simulink model "neckVel"  (Simulink 8.0)
settings: Solver=FixedStepDiscrete  StartTime=0.0  StopTime=inf  FixedStep=Ts  RelTol=1e-3
InitFcn:
  | initBalancingController;
values from neighbouring files (symbols this model uses):
  Gains = [  70    0   0  4]    [initNeckVel.m]
  Impedances = [kImpTorso,kImpArms,kImpArms,kImpLegs,kImpLegs]    [initNeckVel.m]
  Rf = [R, zeros(3,3); zeros(3,3), R]    [initNeckVel.m]
  Ts = 0.01    [initBalancingOptTauQpExtWrenches.m]    (also in initNeckVel.m)
undefined symbols (not defined in the file or in its folder): DiscIntNeverNeededParam
libraries: WBCLibrary x35, simulink x2, dspsigops x2
settings Model: Creator=daniele  LastModifiedBy=daniele
settings DebuggingCC: FcnCallInpInsideContextMsg=EnableAllAsWarning
settings CodeAppCC: CustomSymbolStrType=$N$R$M_T
settings GRTTargetCC: CodeReplacementLibrary=C89/C90 (ANSI)  CombineOutputUpdateFcns=off  GRTInterface=on

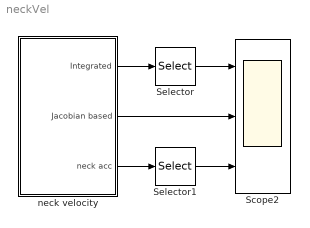
== system neckVel ==
  Scope2 : Scope  NumInputPorts=3
      settings: ShowLegends=on  YMin=-10~-0.035~-0.07  YMax=80~0.04~0.045  SaveName=ScopeData2
  Selector : Selector  InputPortWidth=6  IndexOptions=Index vector (dialog)  Indices=[1:3]  OutputSizes=1
  Selector1 : Selector  InputPortWidth=6  IndexOptions=Index vector (dialog)  Indices=[1:3]  OutputSizes=1
  neck velocity : Subsystem  mask{robotName='iCubGenova01', localName='simulink', Ts=Ts}
      mask prompts: robotName "Robot name"; localName "Local name"
  wires:
  neck velocity/1(Integrated) -> Selector/1
  neck velocity/2(Jacobian based) -> Scope2/2
  Selector/1 -> Scope2/1
  neck velocity/3(neck acc) -> Selector1/1
  Selector1/1 -> Scope2/3

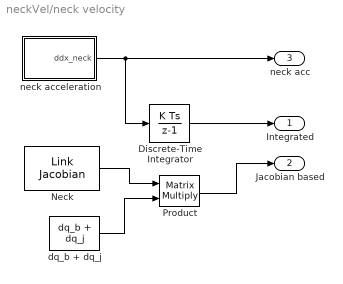
== system neckVel/neck velocity ==
  Discrete-Time Integrator : DiscreteIntegrator  InitialCondition=[0 0 0 0 0 0]  SampleTime=Ts  ICPrevOutput=DiscIntNeverNeededParam  ICPrevScaledInput=DiscIntNeverNeededParam
  Neck : WBCLibrary/wholeBodyModel/Jacobians/Link Jacobian  robotname=robotName  localname=localName  link=chest
  Product : Product  Multiplication=Matrix(*)  SampleTime=Ts  RndMeth=Zero
  dq_b + dq_j : WBCLibrary/wholeBodyStates/dq_b + dq_j  robotName=robotName  localName=localName  Ts=Ts
  neck acceleration : Subsystem  mask{robotName=robotName, localName=localName, Ts=0.010}
      mask prompts: robotName "Robot name"; localName "Local name"
  Integrated : Outport
  Jacobian based : Outport  Port=2
  neck acc : Outport  Port=3
  wires:
  dq_b + dq_j/1 -> Product/2
  Neck/1 -> Product/1
  Product/1 -> Jacobian based/1
  neck acceleration/1(ddx_neck) -> neck acc/1, Discrete-Time Integrator/1
  Discrete-Time Integrator/1 -> Integrated/1

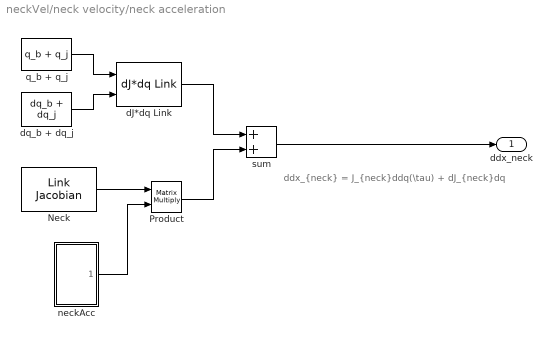
== system neckVel/neck velocity/neck acceleration ==
  note: ddx_{neck} = J_{neck}ddq(\tau) + dJ_{neck}dq
  Neck : WBCLibrary/wholeBodyModel/Jacobians/Link Jacobian  robotname=robotName  localname=localName  link=l_sole
  Product : Product  Multiplication=Matrix(*)  RndMeth=Zero
  dJ*dq Link : WBCLibrary/wholeBodyModel/Dynamics/dJ*dq Link  val=19  robotName=robotName  localName=localName  link=l_sole
  dq_b + dq_j : WBCLibrary/wholeBodyStates/dq_b + dq_j  robotName=robotName  localName=localName  Ts=Ts
  neckAcc : Subsystem  mask{robotName=robotName, Ts=Ts, localName=localName}
      mask prompts: robotName "robot name"; localName "module name"
  q_b + q_j : WBCLibrary/wholeBodyStates/q_b + q_j  robotName=robotName  localName=localName  Ts=Ts
  sum : Sum  SampleTime=Ts
  ddx_neck : Outport
  wires:
  dJ*dq Link/1 -> sum/1
  sum/1 -> ddx_neck/1
  q_b + q_j/1 -> dJ*dq Link/1
  neckAcc/1(ddq(tau)) -> Product/2
  Product/1 -> sum/2
  Neck/1 -> Product/1
  dq_b + dq_j/1 -> dJ*dq Link/2

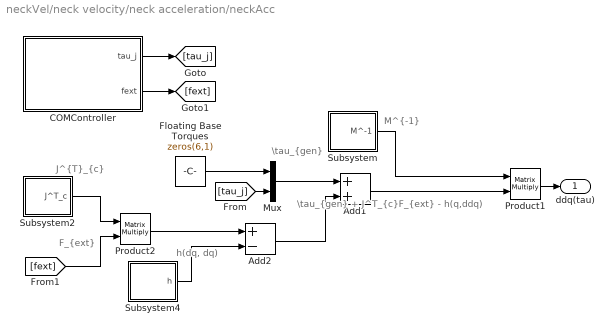
== system neckVel/neck velocity/neck acceleration/neckAcc ==
  note: \tau_{gen} + J^T_{c}F_{ext} - h(q,ddq)
  note: h(dq, dq)
  note: J^{T}_{c}
  note: M^{-1}
  note: F_{ext}
  note: \tau_{gen}
  Add1 : Sum  SampleTime=Ts
  Add2 : Sum  Inputs=+-  SampleTime=Ts
  COMController : Subsystem
  Floating Base Torques : Constant  Value=zeros(6,1)  SampleTime=Ts
  Mux : Mux  Inputs=2
  Product1 : Product  Multiplication=Matrix(*)  SampleTime=Ts
  Product2 : Product  Multiplication=Matrix(*)  SampleTime=Ts
  Subsystem : Subsystem
  Subsystem2 : Subsystem
  Subsystem4 : Subsystem
  ddq(tau) : Outport
  wires:
  Subsystem2/1(J^T_c) -> Product2/1
  [fext] -> Product2/2
  Product2/1 -> Add2/1
  Product1/1 -> ddq(tau)/1
  Add2/1 -> Add1/2
  Subsystem/1(M^-1) -> Product1/1
  Subsystem4/1(h) -> Add2/2
  Add1/1 -> Product1/2
  COMController/1(tau_j) -> [tau_j]
  COMController/2(fext) -> [fext]
  Floating Base Torques/1 -> Mux/1
  [tau_j] -> Mux/2
  Mux/1 -> Add1/1

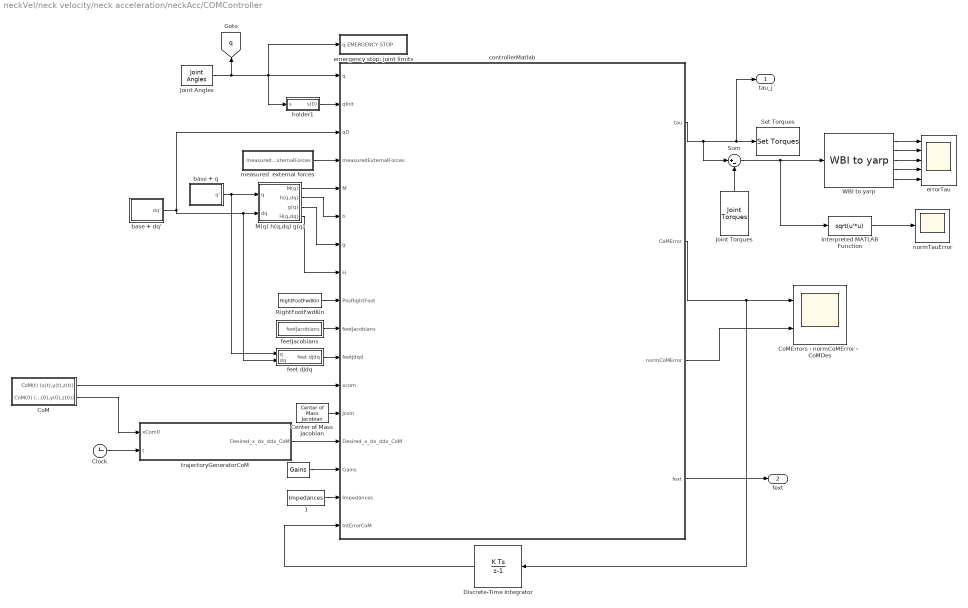
== system neckVel/neck velocity/neck acceleration/neckAcc/COMController ==
  "    " : Constant  Value=Gains
  "    1" : Constant  Value=Impedances
  Center of Mass Jacobian : WBCLibrary/wholeBodyModel/Jacobians/Center of Mass Jacobian  robotName=robotName  localName=localName
  Clock : Clock
  "CoM " : Subsystem
  "CoMErrors - normCoMError -   CoMDes " : Scope  NumInputPorts=2
      settings: ShowLegends=on  TimeRange=35  YMin=-0.1~0  YMax=0.04000000000000001~0.007  SaveName=CoMErrors
  Discrete-Time Integrator : DiscreteIntegrator  InitialCondition=[0 0 0]  SampleTime=Ts  ICPrevOutput=DiscIntNeverNeededParam  ICPrevScaledInput=DiscIntNeverNeededParam
  Interpreted MATLAB Function : MATLABFcn  MATLABFcn=sqrt(u'*u)
  Joint Angles : WBCLibrary/wholeBodyStates/Joint Angles  robotName=robotName  localName=localName
  Joint Torques : WBCLibrary/wholeBodyStates/Joint Torques  robotName=robotName  localName=localName
  M(q) h(q,dq) g(q) : Subsystem
  RightFootFwdKin : WBCLibrary/wholeBodyModel/Forward Kinematics/RightFootFwdKin  robotName=robotName  localName=localName
  Set Torques : WBCLibrary/wholeBodyActuators/Set Torques  val=6  robotName=robotName  localName=localName
  Sum : Sum  Inputs=|+-
  WBI to yarp : WBCLibrary/Utilities/WBI to yarp
  base + dq' : Subsystem
  base + q : Subsystem
  controllerMatlab : MATLAB Function  TreatAsAtomicUnit=on
  emergency stop: joint limits : Subsystem
  errorTau : Scope  NumInputPorts=5
      settings: TimeRange=20  YMin=-12~-5~-5~-5~-5  YMax=6~5~5~5~5
  feet dJdq : Subsystem
  feetJacobians : Subsystem
  holder1 : Subsystem
  measured  external forces : Subsystem
  normTauError : Scope
      settings: TimeRange=80  YMin=0  YMax=60  SaveName=normTauError
  trajectoryGeneratorCoM : MATLAB Function  TreatAsAtomicUnit=on
  tau_j : Outport
  fext : Outport  Port=2
  tag scope: q=global
  wires:
  "    "/1 -> controllerMatlab/15(Gains)
  trajectoryGeneratorCoM/1(Desired_x_dx_ddx_CoM) -> controllerMatlab/14(Desired_x_dx_ddx_CoM)
  Clock/1 -> trajectoryGeneratorCoM/2(t)
  "CoM "/2(CoM(0) (x(0),y(0),z(0))) -> trajectoryGeneratorCoM/1(xCom0)
  RightFootFwdKin/1 -> controllerMatlab/9(PosRightFoot)
  Discrete-Time Integrator/1 -> controllerMatlab/17(IntErrorCoM)
  base + q/1(q') -> feet dJdq/1(q), M(q) h(q,dq) g(q)/1(q)
  base + dq'/1(dq') -> feet dJdq/2(dq), M(q) h(q,dq) g(q)/2(dq), controllerMatlab/3(qD)
  Joint Angles/1 -> [q], emergency stop: joint limits/1(q EMERGENCY STOP), holder1/1(s), controllerMatlab/1(q)
  controllerMatlab/2(CoMError) -> Discrete-Time Integrator/1, "CoMErrors - normCoMError -   CoMDes "/1
  controllerMatlab/3(normCoMError) -> "CoMErrors - normCoMError -   CoMDes "/2
  "    1"/1 -> controllerMatlab/16(Impedances)
  measured  external forces/1(measuredExternalForces) -> controllerMatlab/4(measuredExternalForces)
  Joint Torques/1 -> Sum/2
  Interpreted MATLAB Function/1 -> normTauError/1
  Sum/1 -> WBI to yarp/1, Interpreted MATLAB Function/1
  WBI to yarp/1 -> errorTau/1
  WBI to yarp/2 -> errorTau/2
  WBI to yarp/3 -> errorTau/3
  WBI to yarp/4 -> errorTau/4
  WBI to yarp/5 -> errorTau/5
  M(q) h(q,dq) g(q)/1(M(q)) -> controllerMatlab/5(M)
  M(q) h(q,dq) g(q)/2(h(q,dq)) -> controllerMatlab/6(h)
  M(q) h(q,dq) g(q)/3(g(q)) -> controllerMatlab/7(g)
  "CoM "/1(CoM(t) (x(t),y(t),z(t))) -> controllerMatlab/12(xcom)
  M(q) h(q,dq) g(q)/4(H(q,dq)) -> controllerMatlab/8(H)
  Center of Mass Jacobian/1 -> controllerMatlab/13(Jcom)
  feetJacobians/1(feetJacobians) -> controllerMatlab/10(feetJacobians)
  feet dJdq/1(feet dJdq) -> controllerMatlab/11(feetJdqd)
  holder1/1(s(0)) -> controllerMatlab/2(qInit)
  controllerMatlab/1(tau) -> tau_j/1, Set Torques/1, Sum/1
  controllerMatlab/4(fext) -> fext/1

== system neckVel/neck velocity/neck acceleration/neckAcc/Subsystem ==
  Inv(M) : MATLABFcn  MATLABFcn=inv(u)  Output1D=off  SampleTime=Ts
  massMatrix : WBCLibrary/wholeBodyModel/Dynamics/massMatrix  val=8  robotname=robotName  localname=localName
  q_b + q_j : WBCLibrary/wholeBodyStates/q_b + q_j  robotName=robotName  localName=localName  Ts=Ts
  M^-1 : Outport
  wires:
  q_b + q_j/1 -> massMatrix/1
  Inv(M)/1 -> M^-1/1
  massMatrix/1 -> Inv(M)/1

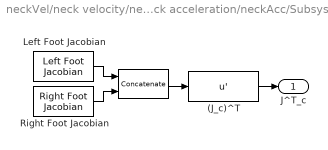
== system neckVel/neck velocity/neck acceleration/neckAcc/Subsystem2 ==
  " " : Concatenate  Mode=Multidimensional array
  (J_c)^T : MATLABFcn  MATLABFcn=u'  Output1D=off  SampleTime=Ts
  Left Foot Jacobian : WBCLibrary/wholeBodyModel/Jacobians/Left Foot Jacobian  robotName=robotName  localName=localName
  Right Foot Jacobian : WBCLibrary/wholeBodyModel/Jacobians/Right Foot Jacobian  robotName=robotName  localName=localName
  J^T_c : Outport
  wires:
  (J_c)^T/1 -> J^T_c/1
  " "/1 -> (J_c)^T/1
  Right Foot Jacobian/1 -> " "/2
  Left Foot Jacobian/1 -> " "/1

== system neckVel/neck velocity/neck acceleration/neckAcc/Subsystem4 ==
  computeh : WBCLibrary/wholeBodyModel/Dynamics/computeh  val=7  robotname=robotName  localname=localName
  dq_b + dq_j : WBCLibrary/wholeBodyStates/dq_b + dq_j  robotName=robotName  localName=localName  Ts=Ts
  q_b + q_j : WBCLibrary/wholeBodyStates/q_b + q_j  robotName=robotName  localName=localName  Ts=Ts
  h : Outport
  wires:
  computeh/1 -> h/1
  q_b + q_j/1 -> computeh/1
  dq_b + dq_j/1 -> computeh/2

== system neckVel/neck velocity/neck acceleration/neckAcc/COMController/CoM  ==
  "COMFwdKin " : WBCLibrary/wholeBodyModel/Forward Kinematics/COMFwdKin   robotName=robotName  localName=localName
  "CoM6D ->  CoMXYZ" : Selector  InputPortWidth=7  IndexOptions=Index vector (dialog)  Indices=[1 2 3]  OutputSizes=1
  holder1 : Subsystem
  CoM(t) (x(t),y(t),z(t)) : Outport
  CoM(0) (x(0),y(0),z(0)) : Outport  Port=2
  wires:
  "COMFwdKin "/1 -> "CoM6D ->  CoMXYZ"/1
  "CoM6D ->  CoMXYZ"/1 -> holder1/1(s), CoM(t) (x(t),y(t),z(t))/1
  holder1/1(s(0)) -> CoM(0) (x(0),y(0),z(0))/1

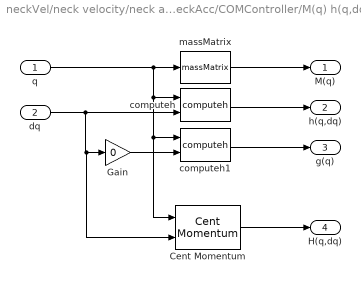
== system neckVel/neck velocity/neck acceleration/neckAcc/COMController/M(q) h(q,dq) g(q) ==
  q : Inport
  dq : Inport  Port=2
  Cent Momentum : WBCLibrary/wholeBodyModel/Dynamics/Cent Momentum  robotName=robotName  localName=localName
  Gain : Gain  Gain=0
  computeh : WBCLibrary/wholeBodyModel/Dynamics/computeh  val=7  robotname=robotName  localname=localName
  computeh1 : WBCLibrary/wholeBodyModel/Dynamics/computeh  val=7  robotname=robotName  localname=localName
  massMatrix : WBCLibrary/wholeBodyModel/Dynamics/massMatrix  val=8  robotname=robotName  localname=localName
  M(q) : Outport
  h(q,dq) : Outport  Port=2
  g(q) : Outport  Port=3
  H(q,dq) : Outport  Port=4
  wires:
  Gain/1 -> computeh1/2
  computeh1/1 -> g(q)/1
  computeh/1 -> h(q,dq)/1
  massMatrix/1 -> M(q)/1
  q/1 -> Cent Momentum/1, computeh1/1, computeh/1, massMatrix/1
  dq/1 -> Cent Momentum/2, Gain/1, computeh/2
  Cent Momentum/1 -> H(q,dq)/1

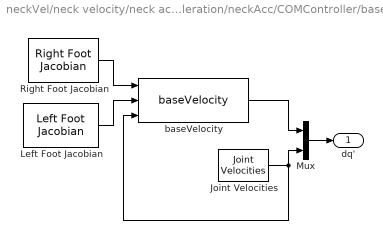
== system neckVel/neck velocity/neck acceleration/neckAcc/COMController/base + dq' ==
  Joint Velocities : WBCLibrary/wholeBodyStates/Joint Velocities  robotName=robotName  localName=localName
  Left Foot Jacobian : WBCLibrary/wholeBodyModel/Jacobians/Left Foot Jacobian  robotName=robotName  localName=localName
  Mux : Mux  Inputs=2
  Right Foot Jacobian : WBCLibrary/wholeBodyModel/Jacobians/Right Foot Jacobian  robotName=robotName  localName=localName
  baseVelocity : WBCLibrary/Utilities/baseVelocity
  dq' : Outport
  wires:
  Left Foot Jacobian/1 -> baseVelocity/2
  Right Foot Jacobian/1 -> baseVelocity/1
  baseVelocity/1 -> Mux/1
  Joint Velocities/1 -> baseVelocity/3, Mux/2
  Mux/1 -> dq'/1

== system neckVel/neck velocity/neck acceleration/neckAcc/COMController/base + q ==
  Constant1 : Constant  Value=zeros(16,1)
  Mux : Mux  Inputs=2
  q' : Outport
  wires:
  Mux/1 -> q'/1
  [q] -> Mux/2
  Constant1/1 -> Mux/1

== system neckVel/neck velocity/neck acceleration/neckAcc/COMController/emergency stop: joint limits ==
  q EMERGENCY STOP : Inport
  Assertion : Assertion  Enabled=on
  Joint Limits1 : WBCLibrary/wholeBodyModel/Joint Limits  robotName=robotName  localName=localName
  MATLAB Function : MATLAB Function  TreatAsAtomicUnit=on
  index1 : Constant  Value=0.01  VectorParams1D=off
  wires:
  Joint Limits1/1 -> MATLAB Function/1(umin)
  Joint Limits1/2 -> MATLAB Function/2(umax)
  index1/1 -> MATLAB Function/4(tol)
  q EMERGENCY STOP/1 -> MATLAB Function/3(u)
  MATLAB Function/1(inRange) -> Assertion/1

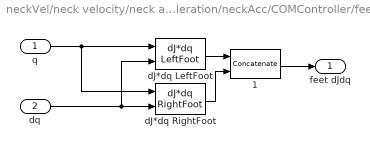
== system neckVel/neck velocity/neck acceleration/neckAcc/COMController/feet dJdq ==
  q : Inport
  dq : Inport  Port=2
  " 1" : Concatenate  Mode=Multidimensional array
  dJ*dq LeftFoot : WBCLibrary/wholeBodyModel/Dynamics/dJ*dq LeftFoot  val=9  robotName=robotName  localName=localName
  dJ*dq RightFoot : WBCLibrary/wholeBodyModel/Dynamics/dJ*dq RightFoot  val=9  robotName=robotName  localName=localName
  feet dJdq : Outport
  wires:
  dJ*dq LeftFoot/1 -> " 1"/1
  dJ*dq RightFoot/1 -> " 1"/2
  " 1"/1 -> feet dJdq/1
  q/1 -> dJ*dq RightFoot/1, dJ*dq LeftFoot/1
  dq/1 -> dJ*dq LeftFoot/2, dJ*dq RightFoot/2

== system neckVel/neck velocity/neck acceleration/neckAcc/COMController/feetJacobians ==
  " " : Concatenate  Mode=Multidimensional array
  Left Foot Jacobian : WBCLibrary/wholeBodyModel/Jacobians/Left Foot Jacobian  robotName=robotName  localName=localName
  Right Foot Jacobian : WBCLibrary/wholeBodyModel/Jacobians/Right Foot Jacobian  robotName=robotName  localName=localName
  feetJacobians : Outport
  wires:
  Left Foot Jacobian/1 -> " "/1
  Right Foot Jacobian/1 -> " "/2
  " "/1 -> feetJacobians/1

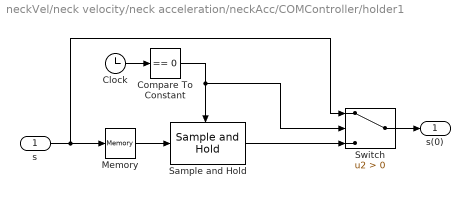
== system neckVel/neck velocity/neck acceleration/neckAcc/COMController/holder1 ==
  s : Inport
  Clock : Clock
  Compare To Constant : simulink/Logic and Bit Operations/Compare To Constant  relop===  const=0  OutDataTypeStr=boolean
  Memory : Memory
  Sample and Hold : dspsigops/Sample and Hold  trig=Falling edge  initCond=0  latchinput=off
  Switch : Switch  Criteria=u2 > Threshold
  s(0) : Outport
  wires:
  s/1 -> Switch/1, Memory/1
  Clock/1 -> Compare To Constant/1
  Compare To Constant/1 -> Sample and Hold/Trigger, Switch/2
  Sample and Hold/1 -> Switch/3
  Switch/1 -> s(0)/1
  Memory/1 -> Sample and Hold/1

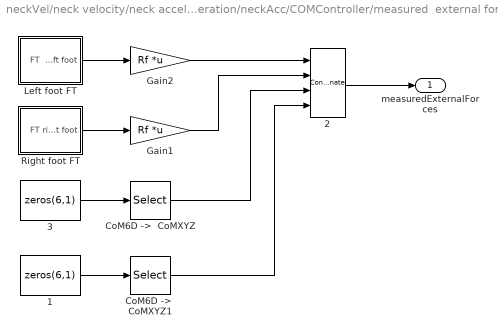
== system neckVel/neck velocity/neck acceleration/neckAcc/COMController/measured  external forces ==
  "    1" : Constant  Value=zeros(6,1)
  "    3" : Constant  Value=zeros(6,1)
  " 2" : Concatenate  NumInputs=4  Mode=Multidimensional array
  "CoM6D ->  CoMXYZ" : Selector  InputPortWidth=6  IndexOptions=Index vector (dialog)  Indices=[1 2 3]  OutputSizes=1
  "CoM6D ->  CoMXYZ1" : Selector  InputPortWidth=6  IndexOptions=Index vector (dialog)  Indices=[1 2 3]  OutputSizes=1
  Gain1 : Gain  Gain=Rf  Multiplication=Matrix(K*u)
  Gain2 : Gain  Gain=Rf  Multiplication=Matrix(K*u)
  Left foot FT : Subsystem
  Right foot FT : Subsystem
  measuredExternalForces : Outport
  wires:
  Right foot FT/1(FT right foot) -> Gain1/1
  Left foot FT/1(FT  left foot) -> Gain2/1
  Gain2/1 -> " 2"/1
  Gain1/1 -> " 2"/2
  " 2"/1 -> measuredExternalForces/1
  "    3"/1 -> "CoM6D ->  CoMXYZ"/1
  "    1"/1 -> "CoM6D ->  CoMXYZ1"/1
  "CoM6D ->  CoMXYZ"/1 -> " 2"/3
  "CoM6D ->  CoMXYZ1"/1 -> " 2"/4

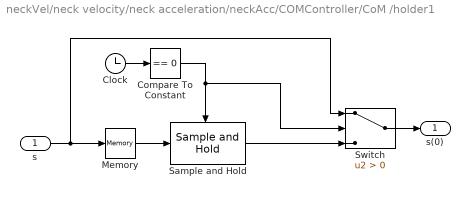
== system neckVel/neck velocity/neck acceleration/neckAcc/COMController/CoM /holder1 ==
  s : Inport
  Clock : Clock
  Compare To Constant : simulink/Logic and Bit Operations/Compare To Constant  relop===  const=0  OutDataTypeStr=boolean
  Memory : Memory
  Sample and Hold : dspsigops/Sample and Hold  trig=Falling edge  initCond=0  latchinput=off
  Switch : Switch  Criteria=u2 > Threshold
  s(0) : Outport
  wires:
  s/1 -> Switch/1, Memory/1
  Clock/1 -> Compare To Constant/1
  Compare To Constant/1 -> Sample and Hold/Trigger, Switch/2
  Sample and Hold/1 -> Switch/3
  Switch/1 -> s(0)/1
  Memory/1 -> Sample and Hold/1

== system neckVel/neck velocity/neck acceleration/neckAcc/COMController/measured  external forces/Left foot FT ==
  Mux : Mux  Inputs=6
  yarp read : WBCLibrary/Utilities/yarp read  from='/wholeBodyDyanmicsTree/left_leg/endEffectorWrench:o'  to='...'  num=6
  FT  left foot : Outport
  wires:
  yarp read/1 -> Mux/1
  yarp read/2 -> Mux/2
  yarp read/3 -> Mux/3
  yarp read/4 -> Mux/4
  yarp read/5 -> Mux/5
  yarp read/6 -> Mux/6
  Mux/1 -> FT  left foot/1

== system neckVel/neck velocity/neck acceleration/neckAcc/COMController/measured  external forces/Right foot FT ==
  Mux : Mux  Inputs=6
  yarp read : WBCLibrary/Utilities/yarp read  from='/wholeBodyDyanmicsTree/right_leg/endEffectorWrench:o'  to='...'  num=6
  FT right foot : Outport
  wires:
  yarp read/1 -> Mux/1
  yarp read/2 -> Mux/2
  yarp read/3 -> Mux/3
  yarp read/4 -> Mux/4
  yarp read/5 -> Mux/5
  yarp read/6 -> Mux/6
  Mux/1 -> FT right foot/1

== matlab function neck velocity/neck acceleration/neckAcc/COMController/trajectoryGeneratorCoM ==
  data: Desired_x_dx_ddx_CoM output double; xCom0 input double; t input double
function Desired_x_dx_ddx_CoM = fcn(xCom0,t)
%#codegen

e3 = [0;1;0];
A = 0.01;
f = 0.15;

xcomDes    = xCom0 + A*sin(2*pi*f*t)*e3;
% xcomDes(1) =  xcomDes(1) + 0.01;
xDcomDes   =         A*2*pi*f*cos(2*pi*f*t)*e3;
xDDcomDes  =        -A*(2*pi*f)^2*sin(2*pi*f*t)*e3;

Desired_x_dx_ddx_CoM = [xcomDes,xDcomDes,xDDcomDes];

== matlab function neck velocity/neck acceleration/neckAcc/COMController/controllerMatlab ==
  data: q input double; qInit input double; qD input double; measuredExternalForces input double; M input double; h input double; g input double; H input double; PosRightFoot input double; feetJacobians input double; tau output double; feetJdqd input double; xcom input double; Jcom input double; Desired_x_dx_ddx_CoM input double; Gains input double; Impedances input double; CoMError output double; IntErrorCoM input double; normCoMError output double; fext output double
function [tau,CoMError,normCoMError,fext] = fcn(q,qInit,qD, measuredExternalForces, M, h, g, H, PosRightFoot, feetJacobians, feetJdqd, xcom,Jcom, Desired_x_dx_ddx_CoM, Gains, Impedances, IntErrorCoM)
%#codegen
PINV_TOL = 1e-5;
gravAcc        = 9.81;

n = 25;
St    = [zeros(6,n);eye(n,n)];

m     = M(1,1);
grav = [zeros(2,1);-m*gravAcc;zeros(3,1)];

% Definition of reference accelerations for CoM and Joints that ensure
% stabilization of desired trajectories xDcomDes and qDes 

xDcom      = Jcom(1:3,:)*qD;
xDDcomStar = Desired_x_dx_ddx_CoM(:,3) - Gains(1)*(xcom - Desired_x_dx_ddx_CoM(:,1)) - Gains(2)*IntErrorCoM - Gains(3)*(xDcom - Desired_x_dx_ddx_CoM(:,2));

Pr =  PosRightFoot(1:3) - xcom; % Application point of the contact force on the right foot w.r.t. CoM

A  = [ eye(3),   zeros(3),eye(3), zeros(3);
      -Sf(xcom),  eye(3), Sf(Pr), eye(3) ];
pinvA = pinv(A, PINV_TOL);
  
HDotDes  = [ m*xDDcomStar ;
            -Gains(4)*H(4:end)]; 

Jc    =   feetJacobians;
           
JcDqD = feetJdqd;
            
desiredFeetContactForces = pinvA*(HDotDes-grav);    

Minv = inv(M);
JcMinv        = Jc*Minv;
PInv_JcMinvSt = pinv(JcMinv*St, PINV_TOL);
N0            = eye(n) - PInv_JcMinvSt*JcMinv*St;

measuredFeetContactForces = desiredFeetContactForces;
fext = measuredFeetContactForces;

tauForDesiredFeetForces = PInv_JcMinvSt*(JcMinv*h - JcDqD - JcMinv*Jc'*measuredFeetContactForces);

tauForImpedenceBehaviour = g(7:end)-Jc(:,7:end)'*measuredFeetContactForces - Impedances.*(q-qInit);

tau = tauForDesiredFeetForces + N0*tauForImpedenceBehaviour;

CoMError    = xcom - Desired_x_dx_ddx_CoM(:,1);
normCoMError  = norm(CoMError);

== matlab function neck velocity/neck acceleration/neckAcc/COMController/emergency stop: joint limits/MATLAB Function ==
  data: umin input double; umax input double; u input double; inRange output double; tol input double
function inRange = checkRange(umin, umax, u, tol)
%#codegen

res = u < umin + tol | u > umax - tol;
res = sum(res);
if res==0
    inRange = 1;
else
    inRange = 0;
    u < umin + tol | u > umax - tol
end
